simulink model "inverseKinematics"  (R2023b)
settings: Solver=VariableStepAuto  StartTime=0.0  StopTime=time(end)  RelTol=1e-3
undefined symbols (not defined in the file or in its folder): DiscIntNeverNeededParam
settings Model: Creator=v4pal  LastModifiedBy=v4pal

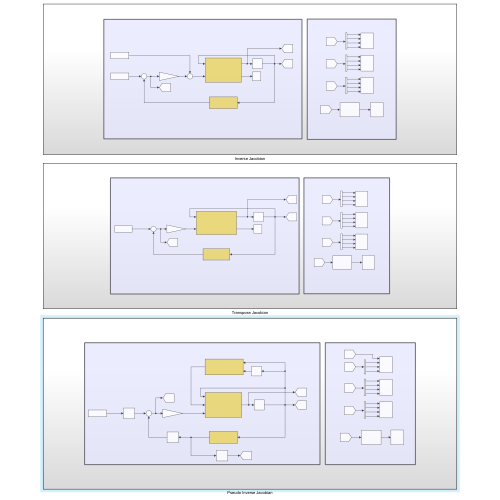
[thumbnail: Simulink's stored preview of the top-level diagram]
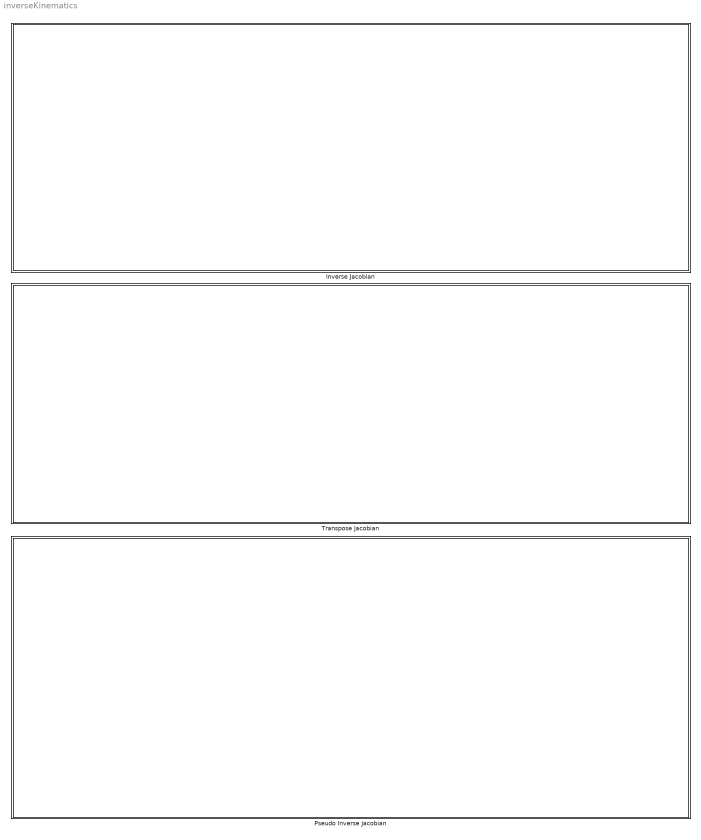
== system inverseKinematics ==
  Inverse Jacobian : Subsystem
  Pseudo Inverse Jacobian : Subsystem
  Transpose Jacobian : Subsystem

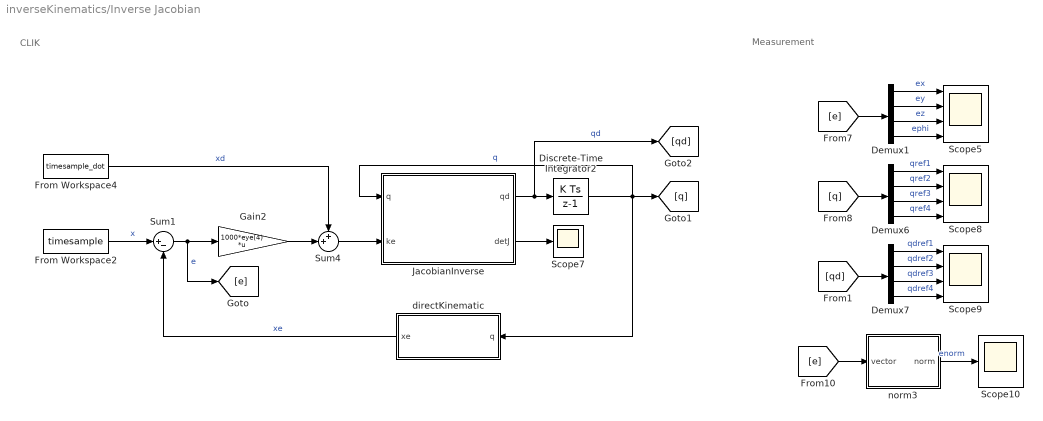
== system inverseKinematics/Inverse Jacobian ==
  note: CLIK
  note: Measurement
  Demux1 : Demux
  Demux6 : Demux
  Demux7 : Demux
  Discrete-Time Integrator2 : DiscreteIntegrator  InitialCondition=[-1.1781; 0.7851; -0.5000; 0.3930]  SampleTime=0.001  ICPrevOutput=DiscIntNeverNeededParam  ICPrevScaledInput=DiscIntNeverNeededParam
  From Workspace2 : FromWorkspace  VariableName=timesample
  From Workspace4 : FromWorkspace  VariableName=timesample_dot
  Gain2 : Gain  Gain=1000*eye(4)  Multiplication=Matrix(K*u)
  JacobianInverse : MATLAB Function  TreatAsAtomicUnit=on
  Scope10 : Scope
  Scope5 : Scope  NumInputPorts=4
  Scope7 : Scope
  Scope8 : Scope  NumInputPorts=4
  Scope9 : Scope  NumInputPorts=4
  Sum1 : Sum  Inputs=|+-
  Sum4 : Sum  Inputs=++|
  directKinematic : MATLAB Function  TreatAsAtomicUnit=on
  norm3 : Subsystem
  wires:
  JacobianInverse/2(detJ) -> Scope7/1
  Sum1/1 -> [e], Gain2/1  "e"
  JacobianInverse/1(qd) -> [qd], Discrete-Time Integrator2/1  "qd"
  From Workspace2/1 -> Sum1/1  "x"
  From Workspace4/1 -> Sum4/1  "xd"
  Discrete-Time Integrator2/1 -> [q], directKinematic/1(q), JacobianInverse/1(q)  "q"
  Sum4/1 -> JacobianInverse/2(ke)
  Gain2/1 -> Sum4/2
  directKinematic/1(xe) -> Sum1/2  "xe"
  Demux1/4 -> Scope5/4  "ephi"
  Demux7/4 -> Scope9/4  "qdref4"
  Demux6/1 -> Scope8/1  "qref1"
  [q] -> Demux6/1
  Demux6/2 -> Scope8/2  "qref2"
  Demux1/3 -> Scope5/3  "ez"
  [e] -> Demux1/1
  Demux1/1 -> Scope5/1  "ex"
  Demux6/3 -> Scope8/3  "qref3"
  Demux7/2 -> Scope9/2  "qdref2"
  [qd] -> Demux7/1
  norm3/1(norm) -> Scope10/1  "enorm"
  Demux6/4 -> Scope8/4  "qref4"
  [e] -> norm3/1(vector)
  Demux7/3 -> Scope9/3  "qdref3"
  Demux1/2 -> Scope5/2  "ey"
  Demux7/1 -> Scope9/1  "qdref1"

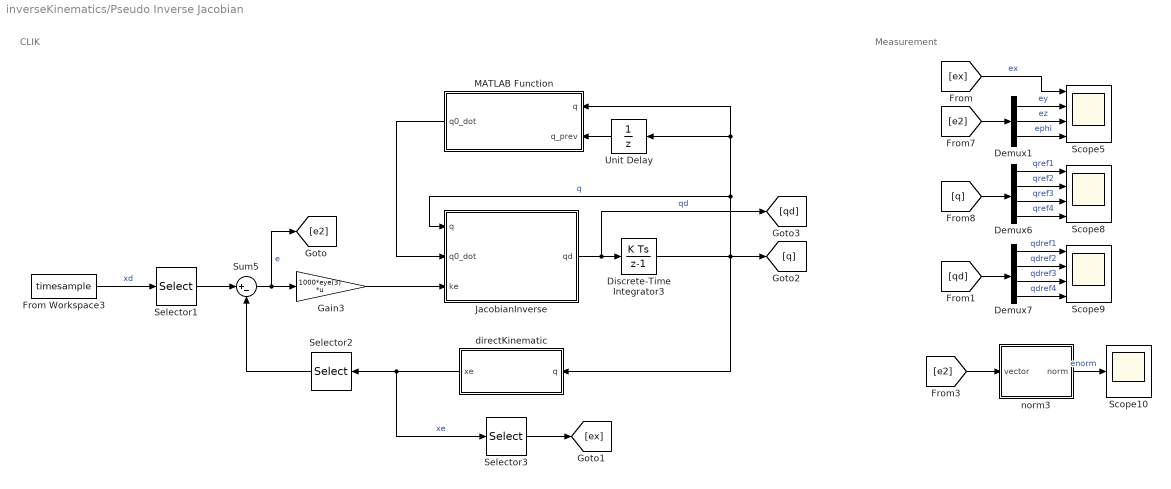
== system inverseKinematics/Pseudo Inverse Jacobian ==
  note: CLIK
  note: Measurement
  Demux1 : Demux  Outputs=3
  Demux6 : Demux
  Demux7 : Demux
  Discrete-Time Integrator3 : DiscreteIntegrator  InitialCondition=[-1.1781; 0.7851; -0.5000; 0.3930]  SampleTime=0.001  ICPrevOutput=DiscIntNeverNeededParam  ICPrevScaledInput=DiscIntNeverNeededParam
  From Workspace3 : FromWorkspace  VariableName=timesample
  Gain3 : Gain  Gain=1000*eye(3)  Multiplication=Matrix(K*u)
  JacobianInverse : MATLAB Function  TreatAsAtomicUnit=on
  MATLAB Function : MATLAB Function  TreatAsAtomicUnit=on
  Scope10 : Scope
  Scope5 : Scope  NumInputPorts=4
  Scope8 : Scope  NumInputPorts=4
  Scope9 : Scope  NumInputPorts=4
  Selector1 : Selector  InputPortWidth=4  IndexOptions=Index vector (dialog)  Indices=[2 3 4]  OutputSizes=1
  Selector2 : Selector  InputPortWidth=4  IndexOptions=Index vector (dialog)  Indices=[2 3 4]  OutputSizes=1
  Selector3 : Selector  InputPortWidth=4  IndexOptions=Index vector (dialog)  Indices=[1]  OutputSizes=1
  Sum5 : Sum  Inputs=|+-
  Unit Delay : UnitDelay  SampleTime=-1  HasFrameUpgradeWarning=on
  directKinematic : MATLAB Function  TreatAsAtomicUnit=on
  norm3 : Subsystem
  wires:
  Sum5/1 -> [e2], Gain3/1  "e"
  Selector1/1 -> Sum5/1
  From Workspace3/1 -> Selector1/1  "xd"
  Selector2/1 -> Sum5/2
  MATLAB Function/1(q0_dot) -> JacobianInverse/2(q0_dot)
  Unit Delay/1 -> MATLAB Function/2(q_prev)
  directKinematic/1(xe) -> Selector3/1, Selector2/1  "xe"
  Gain3/1 -> JacobianInverse/3(ke)
  Discrete-Time Integrator3/1 -> [q], directKinematic/1(q), JacobianInverse/1(q), Unit Delay/1, MATLAB Function/1(q)  "q"
  JacobianInverse/1(qd) -> [qd], Discrete-Time Integrator3/1  "qd"
  Demux1/3 -> Scope5/4  "ephi"
  Demux7/4 -> Scope9/4  "qdref4"
  Demux6/1 -> Scope8/1  "qref1"
  [q] -> Demux6/1
  Demux6/2 -> Scope8/2  "qref2"
  [e2] -> Demux1/1
  Demux6/3 -> Scope8/3  "qref3"
  Demux7/2 -> Scope9/2  "qdref2"
  [qd] -> Demux7/1
  norm3/1(norm) -> Scope10/1  "enorm"
  Demux6/4 -> Scope8/4  "qref4"
  Demux7/3 -> Scope9/3  "qdref3"
  Demux7/1 -> Scope9/1  "qdref1"
  Selector3/1 -> [ex]
  [ex] -> Scope5/1  "ex"
  Demux1/1 -> Scope5/2  "ey"
  Demux1/2 -> Scope5/3  "ez"
  [e2] -> norm3/1(vector)

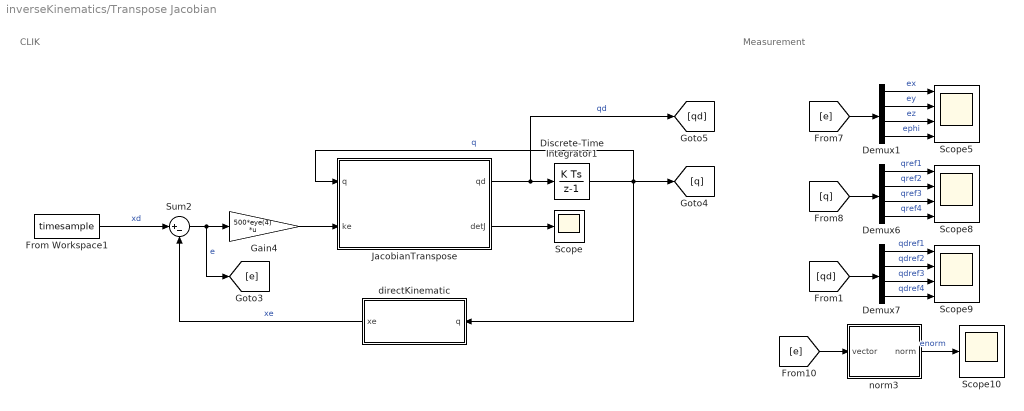
== system inverseKinematics/Transpose Jacobian ==
  note: CLIK
  note: Measurement
  Demux1 : Demux
  Demux6 : Demux
  Demux7 : Demux
  Discrete-Time Integrator1 : DiscreteIntegrator  InitialCondition=[-1.1781; 0.7851; -0.5000; 0.3930]  SampleTime=0.001  ICPrevOutput=DiscIntNeverNeededParam  ICPrevScaledInput=DiscIntNeverNeededParam
  From Workspace1 : FromWorkspace  VariableName=timesample
  Gain4 : Gain  Gain=500*eye(4)  Multiplication=Matrix(K*u)
  JacobianTranspose : MATLAB Function  TreatAsAtomicUnit=on
  Scope : Scope
  Scope10 : Scope
  Scope5 : Scope  NumInputPorts=4
  Scope8 : Scope  NumInputPorts=4
  Scope9 : Scope  NumInputPorts=4
  Sum2 : Sum  Inputs=|+-
  directKinematic : MATLAB Function  TreatAsAtomicUnit=on
  norm3 : Subsystem
  wires:
  Demux1/4 -> Scope5/4  "ephi"
  JacobianTranspose/2(detJ) -> Scope/1
  Gain4/1 -> JacobianTranspose/2(ke)
  Demux7/4 -> Scope9/4  "qdref4"
  directKinematic/1(xe) -> Sum2/2  "xe"
  Sum2/1 -> [e], Gain4/1  "e"
  Demux7/3 -> Scope9/3  "qdref3"
  JacobianTranspose/1(qd) -> [qd], Discrete-Time Integrator1/1  "qd"
  Discrete-Time Integrator1/1 -> [q], directKinematic/1(q), JacobianTranspose/1(q)  "q"
  Demux1/2 -> Scope5/2  "ey"
  From Workspace1/1 -> Sum2/1  "xd"
  [qd] -> Demux7/1
  Demux6/4 -> Scope8/4  "qref4"
  [e] -> norm3/1(vector)
  Demux7/1 -> Scope9/1  "qdref1"
  norm3/1(norm) -> Scope10/1  "enorm"
  Demux7/2 -> Scope9/2  "qdref2"
  [e] -> Demux1/1
  Demux6/2 -> Scope8/2  "qref2"
  Demux1/1 -> Scope5/1  "ex"
  Demux6/3 -> Scope8/3  "qref3"
  Demux1/3 -> Scope5/3  "ez"
  [q] -> Demux6/1
  Demux6/1 -> Scope8/1  "qref1"

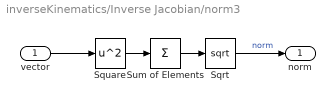
== system inverseKinematics/Inverse Jacobian/norm3 ==
  vector : Inport
  Sqrt : Sqrt
  Square : Math  Operator=square
  Sum of Elements : Sum  Inputs=+
  norm : Outport
  wires:
  Square/1 -> Sum of Elements/1
  Sum of Elements/1 -> Sqrt/1
  vector/1 -> Square/1
  Sqrt/1 -> norm/1  "norm"

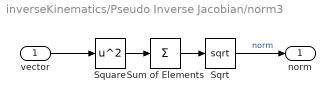
== system inverseKinematics/Pseudo Inverse Jacobian/norm3 ==
  vector : Inport
  Sqrt : Sqrt
  Square : Math  Operator=square
  Sum of Elements : Sum  Inputs=+
  norm : Outport
  wires:
  Square/1 -> Sum of Elements/1
  Sum of Elements/1 -> Sqrt/1
  vector/1 -> Square/1
  Sqrt/1 -> norm/1  "norm"

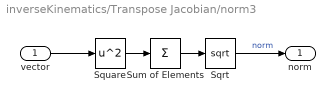
== system inverseKinematics/Transpose Jacobian/norm3 ==
  vector : Inport
  Sqrt : Sqrt
  Square : Math  Operator=square
  Sum of Elements : Sum  Inputs=+
  norm : Outport
  wires:
  Square/1 -> Sum of Elements/1
  Sum of Elements/1 -> Sqrt/1
  vector/1 -> Square/1
  Sqrt/1 -> norm/1  "norm"

== matlab function inverseKinematics/Pseudo Inverse Jacobian/JacobianInverse ==
  data: q input; q0_dot input; ke input; qd output
function qd = inverseJacobian(q, q0_dot, ke) % q = [theta1; theta2]

    % Init the SCARA manipulator parameters
    a1 = .5; a2 = .5;

    theta1 = q(1,:); theta2 = q(2,:);
    %% Geometric Jacobian Matrix
    J = [a1*cos(theta1) + a2*cos(theta1 + theta2), a2*cos(theta1 + theta2), 0, 0;
        0, 0, -1, 0;
        1, 1, 0, -1;];

    % Vx = Jx1 * qd1 + Jx2 * qd2 +Jx3 * qd3;
    % Vy = Jy1 * qd1 + Jy2 * qd2 +Jy3 * qd3;
    % Vz = Jz1 * qd1 + Jz2 * qd2 +Jz3 * qd3;
    
    %J = J(1:2,1:3);
    
    % Calculate the inverse of the Jacobian matrix
    J_pseu = pinv(J);

    % Calculate joint velocities
    qd = J_pseu * ke + (eye(4) - J_pseu*J)*q0_dot;

end

== matlab function inverseKinematics/Inverse Jacobian/directKinematic ==
  data: q input; xe output
function xe = directKinematic(q)
    
    %% Init the SCARA manipulator parameters and Joint variables
    a1 = .5; a2 = .5; d0 = 1;
    theta1 = q(1,:); theta2 = q(2,:); d3 = q(3,:); theta4 = q(4,:);

    %% Forward Kinematics link for the SCARA
    k = [a1*cos(theta1) + a2*cos(theta1 + theta2);
        a1*sin(theta1) + a2*sin(theta1 + theta2);
        d0 - d3;
        theta1 + theta2 - theta4];

    xe = k;

end

== matlab function inverseKinematics/Transpose Jacobian/JacobianTranspose ==
  data: q input; ke input; qd output; detJ output
function [qd, detJ] = JacobianTranspose(q, ke) 

    %% Init the SCARA manipulator parameters and Joint variables
    a1 = .5; a2 = .5;
    theta1 = q(1,:); theta2 = q(2,:);

    %% Geometric Jacobian Matrix
    % J = [a1*cos(theta1) + a2*cos(theta1 + theta2), a2*cos(theta1 + theta2), 0, 0;
    %     0, 0, -1, 0;
    %     1, 1, 0, -1;];

    J = [-a1*sin(theta1) - a2*sin(theta1 + theta2), - a2*sin(theta1 + theta2), 0, 0;
        a1*cos(theta1) + a2*cos(theta1 + theta2), a2*cos(theta1 + theta2), 0, 0;
        0, 0, -1, 0;
        1, 1, 0, -1;];

    % Vx = Jx1 * qd1 + Jx2 * qd2 +Jx3 * qd3;
    % Vy = Jy1 * qd1 + Jy2 * qd2 +Jy3 * qd3;
    % Vz = Jz1 * qd1 + Jz2 * qd2 +Jz3 * qd3;
    
    % J = J(1:3,1:3);
    
    detJ = det(J);

    %% Calculate joint velocities
    qd = J' * ke;

end

== matlab function inverseKinematics/Transpose Jacobian/directKinematic ==
  data: q input; xe output
function xe = directKinematic(q)
    
    %% Init the SCARA manipulator parameters and Joint variables
    a1 = .5; a2 = .5; d0 = 1;
    theta1 = q(1,:); theta2 = q(2,:); d3 = q(3,:); theta4 = q(4,:);

    %% Forward Kinematics link for the SCARA
    k = [a1*cos(theta1) + a2*cos(theta1 + theta2);
        a1*sin(theta1) + a2*sin(theta1 + theta2);
        d0 - d3;
        theta1 + theta2 - theta4;];

    xe = k;

end

== matlab function inverseKinematics/Inverse Jacobian/JacobianInverse ==
  data: q input; ke input; qd output; detJ output
function [qd, detJ] = inverseJacobian(q, ke) % q = [theta1; theta2]

    % Init the SCARA manipulator parameters
    a1 = .5; a2 = .5;

    theta1 = q(1,:); theta2 = q(2,:);
    %% Geometric Jacobian Matrix
    J = [-a1*sin(theta1) - a2*sin(theta1 + theta2), - a2*sin(theta1 + theta2), 0, 0;
        a1*cos(theta1) + a2*cos(theta1 + theta2), a2*cos(theta1 + theta2), 0, 0;
        0, 0, -1, 0;
        1, 1, 0, -1;];

    % Vx = Jx1 * qd1 + Jx2 * qd2 +Jx3 * qd3;
    % Vy = Jy1 * qd1 + Jy2 * qd2 +Jy3 * qd3;
    % Vz = Jz1 * qd1 + Jz2 * qd2 +Jz3 * qd3;
    
    % J = J(1:3,1:3);
    
    detJ = det(J);

    % Calculate joint velocities
    qd = J \ ke;

end

== matlab function inverseKinematics/Pseudo Inverse Jacobian/directKinematic ==
  data: q input; xe output
function xe = directKinematic(q)
    
    %% Init the SCARA manipulator parameters and Joint variables
    a1 = .5; a2 = .5; d0 = 1;
    theta1 = q(1,:); theta2 = q(2,:); d3 = q(3,:); theta4 = q(4,:);

    %% Forward Kinematics link for the SCARA
    k = [a1*cos(theta1) + a2*cos(theta1 + theta2);
        a1*sin(theta1) + a2*sin(theta1 + theta2);
        d0 - d3;
        theta1 + theta2 - theta4;];

    xe = k;

end

== matlab function inverseKinematics/Pseudo Inverse Jacobian/MATLAB Function ==
  data: q input; q0_dot output; q_prev input
function q0_dot = nullVelox(q,q_prev)

    % Init the SCARA manipulator parameters
    a1 = .5; a2 = .5;

    theta1 = q(1,:); theta2 = q(2,:);
    theta1_p = q_prev(1,:); theta2_p = q_prev(2,:);

    %% Geometric Jacobian Matrix
    J = [a1*cos(theta1) + a2*cos(theta1 + theta2), a2*cos(theta1 + theta2), 0, 0;
        0, 0, -1, 0;
        1, 1, 0, -1;];

    J = J(1:3,1:3);

    %% Geometric Jacobian Matrix with q_prev
    J_prev = [a1*cos(theta1_p) + a2*cos(theta1_p + theta2_p), a2*cos(theta1_p + theta2_p), 0, 0;
            0, 0, -1, 0;
            1, 1, 0, -1;];

    J_prev = J(1:3,1:3);

    %% Calculation of q0_dot
    w = sqrt(det(J*J'));
    w_prev = sqrt(det(J_prev*J_prev'));

    k0 = 10;

    dw = w - w_prev;
    dq = q - q_prev;

    q0_dot = k0*(dw/dq)';

    % dw = diff(w);
    % dq = diff(q);
    

end
